simulink model "systema2011a"  (Simulink 7.7)
settings: Solver=ode4  StartTime=0.0  StopTime=20  FixedStep=0.01  RelTol=1e-3
libraries: simulink x11
CloseFcn:
  | rtwprivate ssgencode ModelCloseRequest systema
settings Model: Creator=ece  LastModifiedBy=lenovo
settings DataIOCC: LimitDataPoints=off  SignalLoggingSaveFormat=Dataset  SignalLoggingName=sigsOut
settings OptimizationCC: OptimizeBlockIOStorage=off  BufferReuse=off  ExpressionFolding=off  LocalBlockOutputs=off  InitFltsAndDblsToZero=on
settings DebuggingCC: SaveWithParameterizedLinksMsg=none  SignalResolutionControl=TryResolveAllWithWarning  SolverPrmCheckMsg=none  MultiTaskDSMMsg=warning  MultiTaskCondExecSysMsg=none  FcnCallInpInsideContextMsg=Enable All
settings HardwareCC: TargetUnknown=on
settings CodeAppCC: CustomSymbolStrType=$N$R$M_T
settings GRTTargetCC: TargetFcnLib=ansi_tfl_tmw.mat  TargetFunctionLibrary=C89/C90 (ANSI)  ModelReferenceCompliant=off  MatFileLogging=off

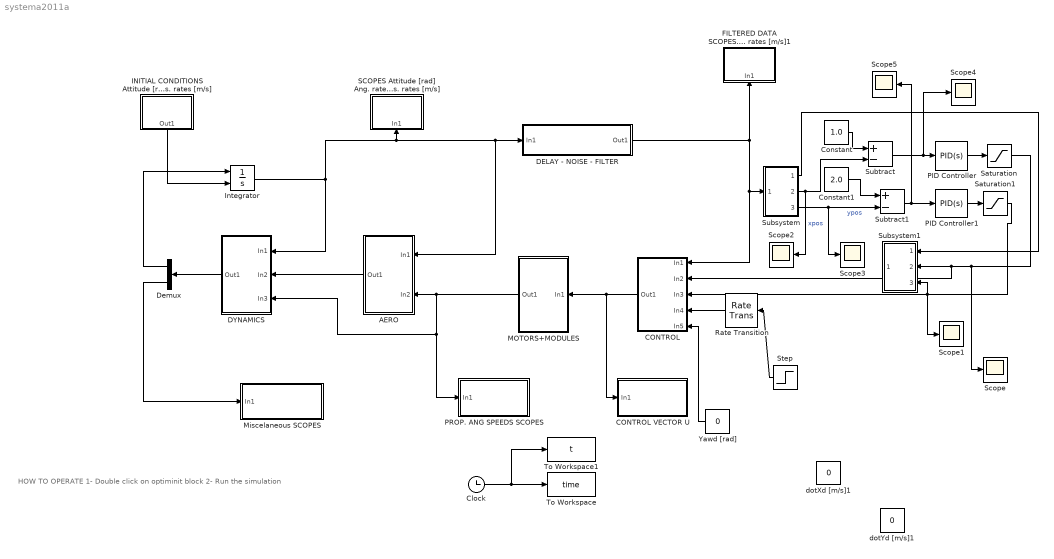
== system systema2011a ==
  note: HOW TO OPERATE
      | 1- Double click on optiminit block
      | 2- Run the simulation
  AERO : Subsystem
  CONTROL : Subsystem
  CONTROL VECTOR U : Subsystem
  Clock : Clock
  Constant : Constant  Value=1.0
  Constant1 : Constant  Value=2.0
  DELAY - NOISE - FILTER : Subsystem
  DYNAMICS : Subsystem
  Demux : Demux  Outputs=2
  FILTERED DATA SCOPES Attitude [rad] Ang. rates [rad/sec] position [m] Pos. rates [m/s]1 : Subsystem
  "INITIAL CONDITIONS Attitude [rad] Ang. rates [rad/sec] position [m] Pos. rates [m/s] " : Subsystem
  Integrator : Integrator  InitialConditionSource=external
  MOTORS+MODULES : Subsystem
  Miscelaneous SCOPES : Subsystem
  PID Controller : simulink/Continuous/PID Controller  Controller=PID  TimeDomain=Continuous-time  SampleTime=-1  IntegratorMethod=Forward Euler  FilterMethod=Forward Euler  Form=Parallel  UseFilter=on  ControllerParametersSource=internal  P=0.8  I=0.2  D=0  N=100  InitialConditionSource=internal  InitialConditionForIntegrator=0  InitialConditionForFilter=0  ExternalReset=none  LimitOutput=off  UpperSaturationLimit=inf  LowerSaturationLimit=-inf  LinearizeAsGain=off  AntiWindupMode=none  Kb=1  TrackingMode=off  Kt=1  PParamMin=[]  PParamMax=[]  IParamMin=[]  IParamMax=[]  DParamMin=[]  DParamMax=[]  NParamMin=[]  NParamMax=[]  KbParamMin=[]  KbParamMax=[]  KtParamMin=[]  KtParamMax=[]  POutMin=[]  POutMax=[]  IOutMin=[]  IOutMax=[]  DOutMin=[]  DOutMax=[]  NOutMin=[]  NOutMax=[]  KbOutMin=[]  KbOutMax=[]  KtOutMin=[]  KtOutMax=[]  IntegratorOutMin=[]  IntegratorOutMax=[]  FilterOutMin=[]  FilterOutMax=[]  SumOutMin=[]  SumOutMax=[]  SumI1OutMin=[]  SumI1OutMax=[]  SumI2OutMin=[]  SumI2OutMax=[]  SumI3OutMin=[]  SumI3OutMax=[]  SumDOutMin=[]  SumDOutMax=[]  SaturationOutMin=[]  SaturationOutMax=[]  IntegratorContinuousStateAttributes=''  IntegratorStateMustResolveToSignalObject=off  IntegratorRTWStateStorageClass=Auto  FilterContinuousStateAttributes=''  FilterStateMustResolveToSignalObject=off  FilterRTWStateStorageClass=Auto  DifferentiatorICPrevScaledInput=0  DifferentiatorOutMin=[]  DifferentiatorOutMax=[]
  PID Controller1 : simulink/Continuous/PID Controller  Controller=PID  TimeDomain=Continuous-time  SampleTime=-1  IntegratorMethod=Forward Euler  FilterMethod=Forward Euler  Form=Parallel  UseFilter=on  ControllerParametersSource=internal  P=1  I=0.2  D=0  N=100  InitialConditionSource=internal  InitialConditionForIntegrator=0  InitialConditionForFilter=0  ExternalReset=none  LimitOutput=off  UpperSaturationLimit=inf  LowerSaturationLimit=-inf  LinearizeAsGain=off  AntiWindupMode=none  Kb=1  TrackingMode=off  Kt=1  PParamMin=[]  PParamMax=[]  IParamMin=[]  IParamMax=[]  DParamMin=[]  DParamMax=[]  NParamMin=[]  NParamMax=[]  KbParamMin=[]  KbParamMax=[]  KtParamMin=[]  KtParamMax=[]  POutMin=[]  POutMax=[]  IOutMin=[]  IOutMax=[]  DOutMin=[]  DOutMax=[]  NOutMin=[]  NOutMax=[]  KbOutMin=[]  KbOutMax=[]  KtOutMin=[]  KtOutMax=[]  IntegratorOutMin=[]  IntegratorOutMax=[]  FilterOutMin=[]  FilterOutMax=[]  SumOutMin=[]  SumOutMax=[]  SumI1OutMin=[]  SumI1OutMax=[]  SumI2OutMin=[]  SumI2OutMax=[]  SumI3OutMin=[]  SumI3OutMax=[]  SumDOutMin=[]  SumDOutMax=[]  SaturationOutMin=[]  SaturationOutMax=[]  IntegratorContinuousStateAttributes=''  IntegratorStateMustResolveToSignalObject=off  IntegratorRTWStateStorageClass=Auto  FilterContinuousStateAttributes=''  FilterStateMustResolveToSignalObject=off  FilterRTWStateStorageClass=Auto  DifferentiatorICPrevScaledInput=0  DifferentiatorOutMin=[]  DifferentiatorOutMax=[]
  PROP. ANG SPEEDS SCOPES : Subsystem
  Rate Transition : RateTransition
  SCOPES Attitude [rad] Ang. rates [rad/sec] position [m] Pos. rates [m/s] : Subsystem
  Saturation : Saturate  UpperLimit=20  LowerLimit=-20
  Saturation1 : Saturate  UpperLimit=20  LowerLimit=-20
  Scope{,1..5} (6 alike) : Scope
      Scope settings: TimeRange=auto  LimitDataPoints=on  MaxDataPoints=5000  SaveToWorkspace=off  SaveName=ScopeData13  YMin=-50  YMax=400  SampleTime=-1
      Scope1 settings: TimeRange=auto  LimitDataPoints=on  MaxDataPoints=5000  SaveToWorkspace=off  SaveName=ScopeData19  YMin=75  YMax=400  SampleTime=-1
      Scope2 settings: TimeRange=auto  LimitDataPoints=on  MaxDataPoints=5000  SaveToWorkspace=off  SaveName=ScopeData28  YMin=-0.16677  YMax=1.5009  SampleTime=-1
      Scope3 settings: TimeRange=auto  LimitDataPoints=on  MaxDataPoints=5000  SaveToWorkspace=off  SaveName=ScopeData29  YMin=-1.59858  YMax=3.92406  SampleTime=-1
      Scope4 settings: TimeRange=auto  LimitDataPoints=on  MaxDataPoints=5000  SaveToWorkspace=off  SaveName=ScopeData30  YMin=75  YMax=400  SampleTime=-1
      Scope5 settings: TimeRange=auto  LimitDataPoints=on  MaxDataPoints=5000  SaveToWorkspace=off  SaveName=ScopeData31  YMin=75  YMax=400  SampleTime=-1
  Step : Step  Time=10  Before=3  After=3.5  SampleTime=0
  Subsystem : Subsystem
  Subsystem1 : Subsystem
  Subtract : Sum  Inputs=+-
  Subtract1 : Sum  Inputs=+-
  To Workspace : ToWorkspace  VariableName=time  SampleTime=-1
  To Workspace1 : ToWorkspace  VariableName=t  SampleTime=-1
  Yawd [rad] : Constant  Value=0
  dotXd [m/s]1 : Constant  Value=0
  dotYd [m/s]1 : Constant  Value=0
  wires:
  Integrator/1 -> SCOPES Attitude [rad] Ang. rates [rad/sec] position [m] Pos. rates [m/s]/1(In1), DELAY - NOISE - FILTER/1(In1), AERO/1(In1), DYNAMICS/1(In1)
  "INITIAL CONDITIONS Attitude [rad] Ang. rates [rad/sec] position [m] Pos. rates [m/s] "/1(Out1) -> Integrator/2
  Clock/1 -> To Workspace/1, To Workspace1/1
  DYNAMICS/1(Out1) -> Demux/1
  Demux/1 -> Integrator/1
  Demux/2 -> Miscelaneous SCOPES/1(In1)
  CONTROL/1(Out1) -> MOTORS+MODULES/1(In1), CONTROL VECTOR U/1(In1)
  Yawd [rad]/1 -> CONTROL/5(In5)
  MOTORS+MODULES/1(Out1) -> AERO/2(In2), DYNAMICS/3(In3), PROP. ANG SPEEDS SCOPES/1(In1)
  AERO/1(Out1) -> DYNAMICS/2(In2)
  DELAY - NOISE - FILTER/1(Out1) -> FILTERED DATA SCOPES Attitude [rad] Ang. rates [rad/sec] position [m] Pos. rates [m/s]1/1(In1), CONTROL/1(In1), Subsystem/1(In1)
  Subtract/1 -> PID Controller/1, Scope4/1
  Subtract1/1 -> PID Controller1/1, Scope5/1
  Subsystem/2(Out3) -> Subtract/2, Scope2/1  "xpos"
  Subsystem/3(Out4) -> Subtract1/2, Scope3/1  "ypos"
  Constant/1 -> Subtract/1
  Constant1/1 -> Subtract1/1
  Subsystem/1(Out2) -> Subsystem1/1(In1)
  PID Controller1/1 -> Saturation1/1
  PID Controller/1 -> Saturation/1
  Saturation/1 -> Scope/1, Subsystem1/2(In2), CONTROL/2(In2)
  Saturation1/1 -> CONTROL/3(In3), Subsystem1/3(In3), Scope1/1
  Rate Transition/1 -> CONTROL/4(In4)
  Step/1 -> Rate Transition/1

== system systema2011a/AERO ==
  In1 : Inport
  In2 : Inport  Port=2
  AERO Attitude [rad] : MATLABFcn  MATLABFcn=aero  OutputDimensions=24
  Mux1 : Mux  Inputs=2
  Out1 : Outport
  wires:
  In1/1 -> Mux1/1
  In2/1 -> Mux1/2
  Mux1/1 -> AERO Attitude [rad]/1
  AERO Attitude [rad]/1 -> Out1/1

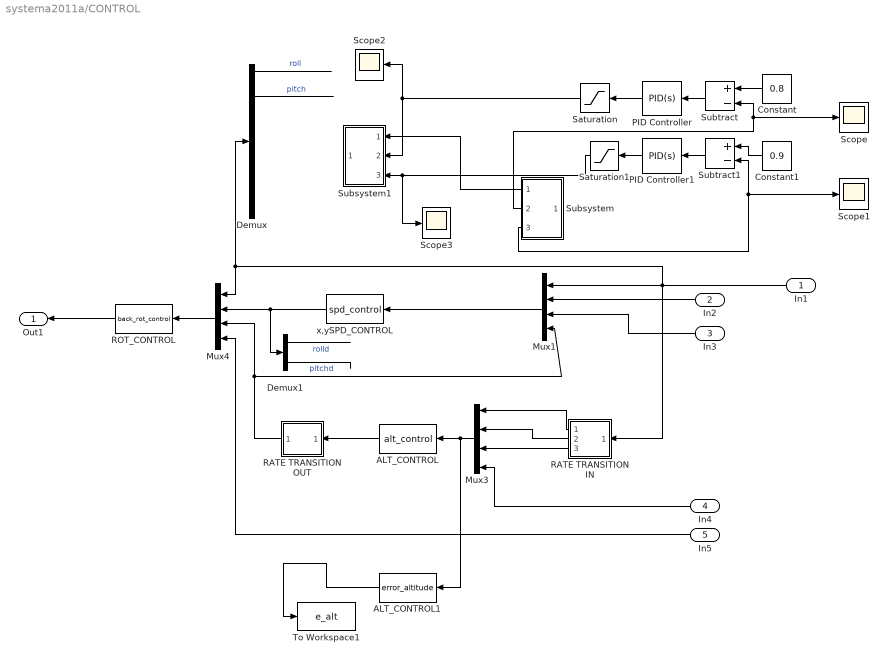
== system systema2011a/CONTROL ==
  In1 : Inport
  In2 : Inport  Port=2
  In3 : Inport  Port=3
  In4 : Inport  Port=4
  In5 : Inport  Port=5
  ALT_CONTROL : MATLABFcn  MATLABFcn=alt_control  OutputDimensions=1  SampleTime=0.05
  ALT_CONTROL1 : MATLABFcn  MATLABFcn=error_altitude  OutputDimensions=1  SampleTime=0.05
  Constant : Constant  Value=0.8
  Constant1 : Constant  Value=0.9
  Demux : Demux  Outputs=12
  Demux1 : Demux  Outputs=2
  Mux1 : Mux
  Mux3 : Mux
  Mux4 : Mux
  PID Controller : simulink/Continuous/PID Controller  Controller=PID  TimeDomain=Continuous-time  SampleTime=-1  IntegratorMethod=Forward Euler  FilterMethod=Forward Euler  Form=Parallel  UseFilter=on  ControllerParametersSource=internal  P=10  I=0.01  D=2  N=100  InitialConditionSource=internal  InitialConditionForIntegrator=0  InitialConditionForFilter=0  ExternalReset=none  LimitOutput=off  UpperSaturationLimit=inf  LowerSaturationLimit=-inf  LinearizeAsGain=off  AntiWindupMode=none  Kb=1  TrackingMode=off  Kt=1  PParamMin=[]  PParamMax=[]  IParamMin=[]  IParamMax=[]  DParamMin=[]  DParamMax=[]  NParamMin=[]  NParamMax=[]  KbParamMin=[]  KbParamMax=[]  KtParamMin=[]  KtParamMax=[]  POutMin=[]  POutMax=[]  IOutMin=[]  IOutMax=[]  DOutMin=[]  DOutMax=[]  NOutMin=[]  NOutMax=[]  KbOutMin=[]  KbOutMax=[]  KtOutMin=[]  KtOutMax=[]  IntegratorOutMin=[]  IntegratorOutMax=[]  FilterOutMin=[]  FilterOutMax=[]  SumOutMin=[]  SumOutMax=[]  SumI1OutMin=[]  SumI1OutMax=[]  SumI2OutMin=[]  SumI2OutMax=[]  SumI3OutMin=[]  SumI3OutMax=[]  SumDOutMin=[]  SumDOutMax=[]  SaturationOutMin=[]  SaturationOutMax=[]  IntegratorContinuousStateAttributes=''  IntegratorStateMustResolveToSignalObject=off  IntegratorRTWStateStorageClass=Auto  FilterContinuousStateAttributes=''  FilterStateMustResolveToSignalObject=off  FilterRTWStateStorageClass=Auto  DifferentiatorICPrevScaledInput=0  DifferentiatorOutMin=[]  DifferentiatorOutMax=[]
  PID Controller1 : simulink/Continuous/PID Controller  Controller=PID  TimeDomain=Continuous-time  SampleTime=-1  IntegratorMethod=Forward Euler  FilterMethod=Forward Euler  Form=Parallel  UseFilter=on  ControllerParametersSource=internal  P=10  I=0.01  D=3  N=100  InitialConditionSource=internal  InitialConditionForIntegrator=0  InitialConditionForFilter=0  ExternalReset=none  LimitOutput=off  UpperSaturationLimit=inf  LowerSaturationLimit=-inf  LinearizeAsGain=off  AntiWindupMode=none  Kb=1  TrackingMode=off  Kt=1  PParamMin=[]  PParamMax=[]  IParamMin=[]  IParamMax=[]  DParamMin=[]  DParamMax=[]  NParamMin=[]  NParamMax=[]  KbParamMin=[]  KbParamMax=[]  KtParamMin=[]  KtParamMax=[]  POutMin=[]  POutMax=[]  IOutMin=[]  IOutMax=[]  DOutMin=[]  DOutMax=[]  NOutMin=[]  NOutMax=[]  KbOutMin=[]  KbOutMax=[]  KtOutMin=[]  KtOutMax=[]  IntegratorOutMin=[]  IntegratorOutMax=[]  FilterOutMin=[]  FilterOutMax=[]  SumOutMin=[]  SumOutMax=[]  SumI1OutMin=[]  SumI1OutMax=[]  SumI2OutMin=[]  SumI2OutMax=[]  SumI3OutMin=[]  SumI3OutMax=[]  SumDOutMin=[]  SumDOutMax=[]  SaturationOutMin=[]  SaturationOutMax=[]  IntegratorContinuousStateAttributes=''  IntegratorStateMustResolveToSignalObject=off  IntegratorRTWStateStorageClass=Auto  FilterContinuousStateAttributes=''  FilterStateMustResolveToSignalObject=off  FilterRTWStateStorageClass=Auto  DifferentiatorICPrevScaledInput=0  DifferentiatorOutMin=[]  DifferentiatorOutMax=[]
  RATE TRANSITION IN : Subsystem
  RATE TRANSITION OUT : Subsystem
  ROT_CONTROL : MATLABFcn  MATLABFcn=back_rot_control  OutputDimensions=6
  Saturation : Saturate  UpperLimit=20  LowerLimit=-20
  Saturation1 : Saturate  UpperLimit=20  LowerLimit=-20
  Scope{,1..3} (4 alike) : Scope
      Scope settings: TimeRange=auto  LimitDataPoints=on  MaxDataPoints=5000  SaveToWorkspace=off  SaveName=ScopeData20  YMin=-0.5  YMax=2  SampleTime=-1
      Scope1 settings: TimeRange=auto  LimitDataPoints=on  MaxDataPoints=5000  SaveToWorkspace=off  SaveName=ScopeData21  YMin=-50  YMax=400  SampleTime=-1
      Scope2 settings: TimeRange=auto  LimitDataPoints=on  MaxDataPoints=5000  SaveToWorkspace=off  SaveName=ScopeData22  YMin=-50  YMax=400  SampleTime=-1
      Scope3 settings: TimeRange=auto  LimitDataPoints=on  MaxDataPoints=5000  SaveToWorkspace=off  SaveName=ScopeData23  YMin=-50  YMax=400  SampleTime=-1
  Subsystem : Subsystem
  Subsystem1 : Subsystem
  Subtract : Sum  Inputs=+-
  Subtract1 : Sum  Inputs=+-
  To Workspace1 : ToWorkspace  VariableName=e_alt  SampleTime=-1
  x,ySPD_CONTROL : MATLABFcn  MATLABFcn=spd_control  OutputDimensions=2
  Out1 : Outport
  wires:
  Mux1/1 -> x,ySPD_CONTROL/1
  ROT_CONTROL/1 -> Out1/1
  In1/1 -> Mux1/1, RATE TRANSITION IN/1(In1), Demux/1, Mux4/1
  In2/1 -> Mux1/2
  x,ySPD_CONTROL/1 -> Demux1/1, Mux4/2
  Mux4/1 -> ROT_CONTROL/1
  ALT_CONTROL/1 -> RATE TRANSITION OUT/1(In1)
  In5/1 -> Mux4/4
  RATE TRANSITION OUT/1(Out1) -> Mux4/3, Mux1/4
  Mux3/1 -> ALT_CONTROL/1, ALT_CONTROL1/1
  RATE TRANSITION IN/1(Out1) -> Mux3/1
  RATE TRANSITION IN/2(Out2) -> Mux3/2
  RATE TRANSITION IN/3(Out3) -> Mux3/3
  In4/1 -> Mux3/4
  In3/1 -> Mux1/3
  ALT_CONTROL1/1 -> To Workspace1/1
  Subtract/1 -> PID Controller/1
  Subtract1/1 -> PID Controller1/1
  Constant/1 -> Subtract/1
  Constant1/1 -> Subtract1/1
  PID Controller1/1 -> Saturation1/1
  PID Controller/1 -> Saturation/1
  Subsystem/1(Out2) -> Subsystem1/1(In1)
  Subsystem/2(Out3) -> Subtract/2, Scope/1
  Subsystem/3(Out4) -> Subtract1/2, Scope1/1
  Saturation/1 -> Subsystem1/2(In2), Scope2/1
  Saturation1/1 -> Subsystem1/3(In3), Scope3/1
  Demux/1 -> ?  "roll"
  Demux/3 -> ?  "pitch"
  Demux1/1 -> ?  "rolld"
  Demux1/2 -> ?  "pitchd"

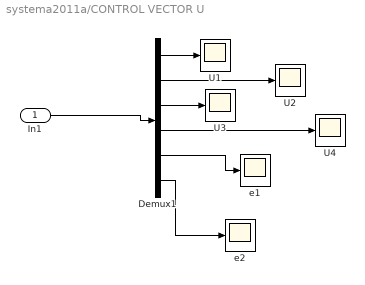
== system systema2011a/CONTROL VECTOR U ==
  In1 : Inport
  Demux1 : Demux  Outputs=6
  U{1..4} (4 alike) : Scope
      U1 settings: TimeRange=3.5  MaxDataPoints=5000  SaveToWorkspace=off  SaveName=ScopeData7  YMin=144.101  YMax=144.104  SampleTime=-1
      U2 settings: TimeRange=auto  MaxDataPoints=5000  SaveToWorkspace=off  SaveName=ScopeData8  YMin=-0.6  YMax=0.4  SampleTime=-1
      U3 settings: TimeRange=auto  MaxDataPoints=5000  SaveToWorkspace=off  SaveName=ScopeData9  YMin=-0.65  YMax=0.35  SampleTime=-1
      U4 settings: TimeRange=auto  MaxDataPoints=5000  SaveToWorkspace=off  SaveName=ScopeData14  YMin=0  YMax=150  SampleTime=-1
  e1 : Scope
      settings: TimeRange=auto  MaxDataPoints=5000  SaveToWorkspace=off  SaveName=ScopeData11  YMin=0  YMax=150  SampleTime=-1
  e2 : Scope
      settings: TimeRange=auto  MaxDataPoints=5000  SaveToWorkspace=off  SaveName=ScopeData12  YMin=0  YMax=150  SampleTime=-1
  wires:
  In1/1 -> Demux1/1
  Demux1/4 -> U4/1
  Demux1/3 -> U3/1
  Demux1/2 -> U2/1
  Demux1/1 -> U1/1
  Demux1/5 -> e1/1
  Demux1/6 -> e2/1

== system systema2011a/DELAY - NOISE - FILTER ==
  In1 : Inport
  DELAYS : Subsystem
  LP FILTER : MATLABFcn  MATLABFcn=sam5_filter  OutputDimensions=12  OutputSignalType=real
  NOISY DATA SCOPES Attitude [rad] Ang. rates [rad/sec] position [m] Pos. rates [m/s]1 : Subsystem
  W. NORMAL NOISE1 : Subsystem
  Out1 : Outport
  wires:
  In1/1 -> DELAYS/1(In1)
  DELAYS/1(Out1) -> NOISY DATA SCOPES Attitude [rad] Ang. rates [rad/sec] position [m] Pos. rates [m/s]1/1(In1), LP FILTER/1
  LP FILTER/1 -> Out1/1

== system systema2011a/DYNAMICS ==
  In1 : Inport
  In2 : Inport  Port=2
  In3 : Inport  Port=3
  DYNAMICS : MATLABFcn  MATLABFcn=dinamica  OutputDimensions=18
  Mux1 : Mux  Inputs=3
  Out1 : Outport
  wires:
  DYNAMICS/1 -> Out1/1
  Mux1/1 -> DYNAMICS/1
  In2/1 -> Mux1/2
  In1/1 -> Mux1/1
  In3/1 -> Mux1/3

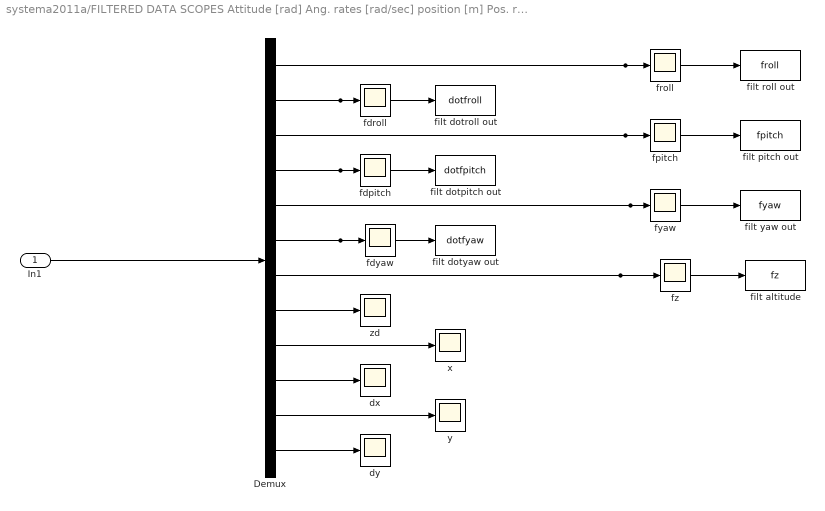
== system systema2011a/FILTERED DATA SCOPES Attitude [rad] Ang. rates [rad/sec] position [m] Pos. rates [m/s]1 ==
  In1 : Inport
  Demux : Demux  Outputs=12
  dx : Scope
      settings: TimeRange=5  MaxDataPoints=5000  SaveToWorkspace=off  SaveName=ScopeData5  YMin=0  YMax=0.009  SampleTime=-1
  dy : Scope
      settings: TimeRange=5  MaxDataPoints=5000  SaveToWorkspace=off  SaveName=ScopeData10  YMin=0  YMax=0.009  SampleTime=-1
  fdpitch : Scope
      settings: TimeRange=auto  MaxDataPoints=5000  SaveToWorkspace=off  SaveName=ScopeData15  YMin=-2250  YMax=2250  SampleTime=-1
  fdroll : Scope
      settings: TimeRange=auto  MaxDataPoints=5000  SaveToWorkspace=off  SaveName=ScopeData14  YMin=-0.25  YMax=-0.05  SampleTime=-1
  fdyaw : Scope
      settings: TimeRange=18  MaxDataPoints=5000  SaveToWorkspace=off  SaveName=ScopeData16  YMin=-200  YMax=200  SampleTime=-1
  filt altitude : ToWorkspace  VariableName=fz  SampleTime=-1
  filt dotpitch out : ToWorkspace  VariableName=dotfpitch  SampleTime=-1
  filt dotroll out : ToWorkspace  VariableName=dotfroll  SampleTime=-1
  filt dotyaw out : ToWorkspace  VariableName=dotfyaw  SampleTime=-1
  filt pitch out : ToWorkspace  VariableName=fpitch  SampleTime=-1
  filt roll out : ToWorkspace  VariableName=froll  SampleTime=-1
  filt yaw out : ToWorkspace  VariableName=fyaw  SampleTime=-1
  fpitch : Scope
      settings: TimeRange=4  MaxDataPoints=5000  SaveToWorkspace=off  YMin=-1  YMax=1  SampleTime=-1
  froll : Scope
      settings: TimeRange=0.25  MaxDataPoints=5000  SaveToWorkspace=off  SaveName=ScopeData  YMin=-1  YMax=1  SampleTime=-1
  fyaw : Scope
      settings: TimeRange=5  MaxDataPoints=5000  SaveToWorkspace=off  SaveName=ScopeData2  YMin=0  YMax=0.22  SampleTime=-1
  fz : Scope
      settings: TimeRange=5  MaxDataPoints=5000  SaveToWorkspace=off  SaveName=ScopeData17  YMin=-0.45  YMax=0.5  SampleTime=-1
  x : Scope
      settings: TimeRange=5  MaxDataPoints=5000  SaveToWorkspace=off  SaveName=ScopeData4  YMin=0  YMax=0.009  SampleTime=-1
  y : Scope
      settings: TimeRange=5  MaxDataPoints=5000  SaveToWorkspace=off  SaveName=ScopeData6  YMin=0  YMax=0.009  SampleTime=-1
  zd : Scope
      settings: TimeRange=10  MaxDataPoints=5000  SaveToWorkspace=off  SaveName=ScopeData18  YMin=-110.5  YMax=-107.25  SampleTime=-1
  wires:
  Demux/1 -> filt roll out/1, froll/1
  Demux/4 -> fdpitch/1, filt dotpitch out/1
  Demux/8 -> zd/1
  Demux/7 -> filt altitude/1, fz/1
  Demux/6 -> fdyaw/1, filt dotyaw out/1
  Demux/2 -> fdroll/1, filt dotroll out/1
  Demux/5 -> filt yaw out/1, fyaw/1
  Demux/3 -> filt pitch out/1, fpitch/1
  In1/1 -> Demux/1
  Demux/9 -> x/1
  Demux/10 -> dx/1
  Demux/11 -> y/1
  Demux/12 -> dy/1

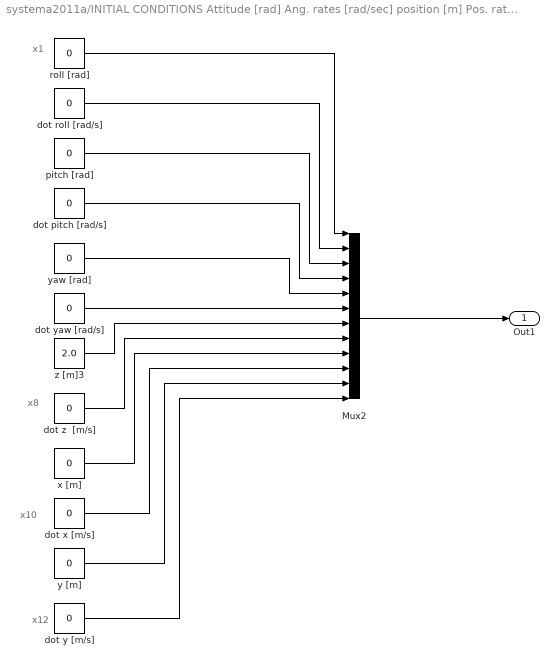
== system systema2011a/INITIAL CONDITIONS Attitude [rad] Ang. rates [rad/sec] position [m] Pos. rates [m/s]  ==
  note: x1
  note: x12
  note: x10
  note: x8
  Mux2 : Mux  Inputs=12
  dot pitch [rad/s] : Constant  Value=0
  dot roll [rad/s] : Constant  Value=0
  dot x [m/s] : Constant  Value=0
  dot y [m/s] : Constant  Value=0
  dot yaw [rad/s] : Constant  Value=0
  dot z  [m/s] : Constant  Value=0
  pitch [rad] : Constant  Value=0
  roll [rad] : Constant  Value=0
  x [m] : Constant  Value=0
  y [m] : Constant  Value=0
  yaw [rad] : Constant  Value=0
  z [m]3 : Constant  Value=2.0
  Out1 : Outport
  wires:
  roll [rad]/1 -> Mux2/1
  dot roll [rad/s]/1 -> Mux2/2
  pitch [rad]/1 -> Mux2/3
  dot pitch [rad/s]/1 -> Mux2/4
  dot yaw [rad/s]/1 -> Mux2/6
  z [m]3/1 -> Mux2/7
  dot z  [m/s]/1 -> Mux2/8
  yaw [rad]/1 -> Mux2/5
  Mux2/1 -> Out1/1
  x [m]/1 -> Mux2/9
  dot x [m/s]/1 -> Mux2/10
  y [m]/1 -> Mux2/11
  dot y [m/s]/1 -> Mux2/12

== system systema2011a/MOTORS+MODULES ==
  In1 : Inport
  Bin2Om : MATLABFcn  MATLABFcn=bin2Om  OutputDimensions=4  OutputSignalType=real
  MOTOR DYNAMICS : Subsystem
  Saturation : Saturate  UpperLimit=125  LowerLimit=10
  U2bin : MATLABFcn  MATLABFcn=U2bin  OutputDimensions=4  OutputSignalType=real
  Out1 : Outport
  wires:
  Bin2Om/1 -> Out1/1
  MOTOR DYNAMICS/1(Out1) -> Bin2Om/1
  U2bin/1 -> Saturation/1
  In1/1 -> U2bin/1
  Saturation/1 -> MOTOR DYNAMICS/1(In1)

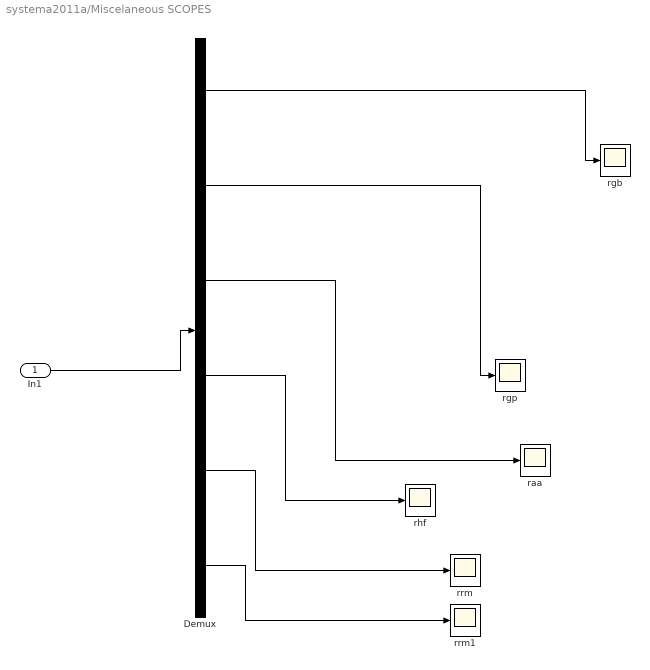
== system systema2011a/Miscelaneous SCOPES ==
  In1 : Inport  PortDimensions=6
  Demux : Demux  Outputs=6
  raa : Scope
      settings: TimeRange=18  MaxDataPoints=5000  SaveToWorkspace=off  SaveName=ScopeData16  YMin=-200  YMax=200  SampleTime=-1
  rgb : Scope
      settings: TimeRange=auto  MaxDataPoints=5000  SaveToWorkspace=off  SaveName=ScopeData14  YMin=-0.25  YMax=-0.05  SampleTime=-1
  rgp : Scope
      settings: TimeRange=auto  MaxDataPoints=5000  SaveToWorkspace=off  SaveName=ScopeData15  YMin=-2250  YMax=2250  SampleTime=-1
  rhf : Scope
      settings: TimeRange=10  MaxDataPoints=5000  SaveToWorkspace=off  SaveName=ScopeData18  YMin=-110.5  YMax=-107.25  SampleTime=-1
  rrm : Scope
      settings: TimeRange=5  MaxDataPoints=5000  SaveToWorkspace=off  SaveName=ScopeData25  YMin=-4.75e-015  YMax=0  SampleTime=-1
  rrm1 : Scope
      settings: TimeRange=5  MaxDataPoints=5000  SaveToWorkspace=off  SaveName=ScopeData3  YMin=-4.75e-015  YMax=0  SampleTime=-1
  wires:
  In1/1 -> Demux/1
  Demux/5 -> rrm/1
  Demux/4 -> rhf/1
  Demux/3 -> raa/1
  Demux/2 -> rgp/1
  Demux/1 -> rgb/1
  Demux/6 -> rrm1/1

== system systema2011a/PROP. ANG SPEEDS SCOPES ==
  In1 : Inport
  Demux1 : Demux
  omega{1..4} (4 alike) : Scope
      omega1 settings: TimeRange=3.5  MaxDataPoints=5000  SaveToWorkspace=off  SaveName=ScopeData7  YMin=144.101  YMax=144.104  SampleTime=-1
      omega2 settings: TimeRange=auto  MaxDataPoints=5000  SaveToWorkspace=off  SaveName=ScopeData8  YMin=142.5  YMax=147.5  SampleTime=-1
      omega3 settings: TimeRange=auto  MaxDataPoints=5000  SaveToWorkspace=off  SaveName=ScopeData9  YMin=0  YMax=150  SampleTime=-1
      omega4 settings: TimeRange=auto  MaxDataPoints=5000  SaveToWorkspace=off  SaveName=ScopeData14  YMin=0  YMax=150  SampleTime=-1
  wires:
  Demux1/1 -> omega1/1
  Demux1/2 -> omega2/1
  Demux1/3 -> omega3/1
  Demux1/4 -> omega4/1
  In1/1 -> Demux1/1

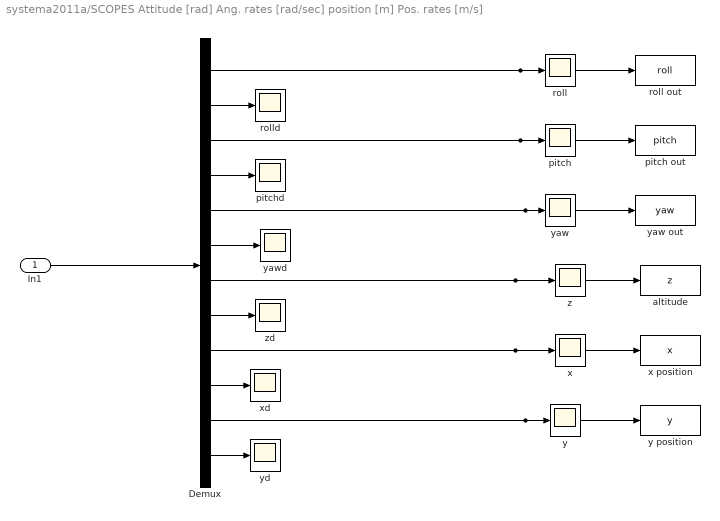
== system systema2011a/SCOPES Attitude [rad] Ang. rates [rad/sec] position [m] Pos. rates [m/s] ==
  In1 : Inport
  Demux : Demux  Outputs=12
  altitude : ToWorkspace  VariableName=z  SampleTime=-1
  pitch : Scope
      settings: TimeRange=4  MaxDataPoints=5000  SaveToWorkspace=off  YMin=-0.08  YMax=0.16  SampleTime=-1
  pitch out : ToWorkspace  VariableName=pitch  SampleTime=-1
  pitchd : Scope
      settings: TimeRange=auto  MaxDataPoints=5000  SaveToWorkspace=off  SaveName=ScopeData15  YMin=-1.75  YMax=1.75  SampleTime=-1
  roll : Scope
      settings: TimeRange=0.25  MaxDataPoints=5000  SaveToWorkspace=off  SaveName=ScopeData  YMin=-0.008  YMax=0.005  SampleTime=-1
  roll out : ToWorkspace  VariableName=roll  SampleTime=-1
  rolld : Scope
      settings: TimeRange=7  MaxDataPoints=5000  SaveToWorkspace=off  SaveName=ScopeData14  YMin=-0.15  YMax=0.125  SampleTime=-1
  x : Scope
      settings: TimeRange=5  MaxDataPoints=5000  SaveToWorkspace=off  SaveName=ScopeData24  YMin=-1  YMax=1  SampleTime=-1
  x position : ToWorkspace  VariableName=x  SampleTime=-1
  xd : Scope
      settings: TimeRange=5  MaxDataPoints=5000  SaveToWorkspace=off  SaveName=ScopeData25  YMin=-4.75e-015  YMax=0  SampleTime=-1
  y : Scope
      settings: TimeRange=5  MaxDataPoints=5000  SaveToWorkspace=off  SaveName=ScopeData26  YMin=-1  YMax=1  SampleTime=-1
  y position : ToWorkspace  VariableName=y  SampleTime=-1
  yaw : Scope
      settings: TimeRange=5  MaxDataPoints=5000  SaveToWorkspace=off  SaveName=ScopeData2  YMin=-175  YMax=0  SampleTime=-1
  yaw out : ToWorkspace  VariableName=yaw  SampleTime=-1
  yawd : Scope
      settings: TimeRange=18  MaxDataPoints=5000  SaveToWorkspace=off  SaveName=ScopeData16  YMin=-0.275  YMax=0.15  SampleTime=-1
  yd : Scope
      settings: TimeRange=5  MaxDataPoints=5000  SaveToWorkspace=off  SaveName=ScopeData27  YMin=-143.75  YMax=-141.75  SampleTime=-1
  z : Scope
      settings: TimeRange=5  MaxDataPoints=5000  SaveToWorkspace=off  SaveName=ScopeData17  YMin=0  YMax=0.009  SampleTime=-1
  zd : Scope
      settings: TimeRange=10  MaxDataPoints=5000  SaveToWorkspace=off  SaveName=ScopeData18  YMin=-110.5  YMax=-107.25  SampleTime=-1
  wires:
  In1/1 -> Demux/1
  Demux/3 -> pitch/1, pitch out/1
  Demux/5 -> yaw/1, yaw out/1
  Demux/2 -> rolld/1
  Demux/6 -> yawd/1
  Demux/7 -> z/1, altitude/1
  Demux/8 -> zd/1
  Demux/9 -> x/1, x position/1
  Demux/11 -> y/1, y position/1
  Demux/12 -> yd/1
  Demux/10 -> xd/1
  Demux/4 -> pitchd/1
  Demux/1 -> roll/1, roll out/1

== system systema2011a/Subsystem ==
  In1 : Inport
  Demux1 : Demux  Outputs=12
  Double click on this for demo.5 : Subsystem
      settings: OpenFcn=optsiminit
      mask Display: disp('optsiminit')
  Mux1 : Mux  Inputs=10
  Out2 : Outport
  Out3 : Outport  Port=2
  Out4 : Outport  Port=3
  wires:
  Demux1/1 -> Mux1/1
  Demux1/2 -> Mux1/2
  Demux1/3 -> Mux1/3
  Demux1/4 -> Mux1/4
  Demux1/5 -> Mux1/5
  Demux1/6 -> Mux1/6
  Demux1/7 -> Mux1/7
  Demux1/8 -> Mux1/8
  Demux1/10 -> Mux1/9
  Demux1/12 -> Mux1/10
  Mux1/1 -> Out2/1
  Demux1/9 -> Out3/1
  Demux1/11 -> Out4/1
  In1/1 -> Demux1/1

== system systema2011a/Subsystem1 ==
  In1 : Inport
  In2 : Inport  Port=2
  In3 : Inport  Port=3
  Demux1 : Demux  Outputs=10
  Mux1 : Mux  Inputs=12
  Out5 : Outport
  wires:
  In1/1 -> Demux1/1
  Demux1/1 -> Mux1/1
  Demux1/2 -> Mux1/2
  Demux1/3 -> Mux1/3
  Demux1/4 -> Mux1/4
  Demux1/5 -> Mux1/5
  Demux1/6 -> Mux1/6
  Demux1/7 -> Mux1/7
  Demux1/8 -> Mux1/8
  Demux1/10 -> Mux1/12
  Demux1/9 -> Mux1/10
  In2/1 -> Mux1/9
  In3/1 -> Mux1/11
  Mux1/1 -> Out5/1

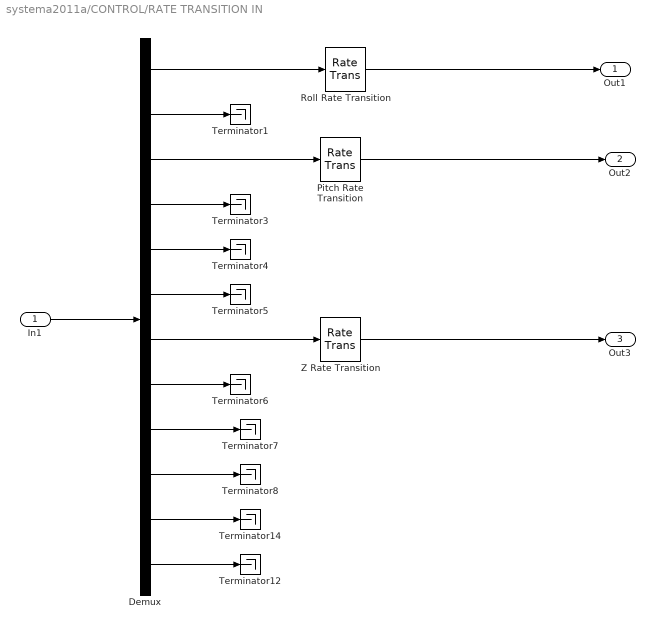
== system systema2011a/CONTROL/RATE TRANSITION IN ==
  In1 : Inport
  Demux : Demux  Outputs=12
  Pitch Rate Transition : RateTransition  Deterministic=off  OutPortSampleTime=50E-3
  Roll Rate Transition : RateTransition  Deterministic=off  OutPortSampleTime=50E-3
  Terminator{1,3..8,12,14} (9 alike) : Terminator
  Z Rate Transition : RateTransition  Deterministic=off  OutPortSampleTime=50E-3
  Out1 : Outport
  Out2 : Outport  Port=2
  Out3 : Outport  Port=3
  wires:
  Demux/7 -> Z Rate Transition/1
  In1/1 -> Demux/1
  Demux/1 -> Roll Rate Transition/1
  Demux/2 -> Terminator1/1
  Demux/3 -> Pitch Rate Transition/1
  Demux/4 -> Terminator3/1
  Demux/5 -> Terminator4/1
  Demux/6 -> Terminator5/1
  Demux/9 -> Terminator7/1
  Demux/10 -> Terminator8/1
  Demux/11 -> Terminator14/1
  Demux/12 -> Terminator12/1
  Demux/8 -> Terminator6/1
  Roll Rate Transition/1 -> Out1/1
  Pitch Rate Transition/1 -> Out2/1
  Z Rate Transition/1 -> Out3/1

== system systema2011a/CONTROL/RATE TRANSITION OUT ==
  In1 : Inport
  Rate Transition1 : RateTransition  Deterministic=off
  Out1 : Outport
  wires:
  In1/1 -> Rate Transition1/1
  Rate Transition1/1 -> Out1/1

== system systema2011a/CONTROL/Subsystem ==
  In1 : Inport
  Demux1 : Demux  Outputs=12
  Double click on this for demo.5 : Subsystem
      settings: OpenFcn=optsiminit
      mask Display: disp('optsiminit')
  Mux1 : Mux  Inputs=10
  Out2 : Outport
  Out3 : Outport  Port=2
  Out4 : Outport  Port=3
  wires:
  Demux1/1 -> Mux1/1
  Demux1/2 -> Mux1/2
  Demux1/3 -> Mux1/3
  Demux1/4 -> Mux1/4
  Demux1/5 -> Mux1/5
  Demux1/6 -> Mux1/6
  Demux1/7 -> Mux1/7
  Demux1/8 -> Mux1/8
  Demux1/10 -> Mux1/9
  Demux1/12 -> Mux1/10
  Mux1/1 -> Out2/1
  Demux1/9 -> Out3/1
  Demux1/11 -> Out4/1
  In1/1 -> Demux1/1

== system systema2011a/CONTROL/Subsystem1 ==
  In1 : Inport
  In2 : Inport  Port=2
  In3 : Inport  Port=3
  Demux1 : Demux  Outputs=10
  Mux1 : Mux  Inputs=12
  Out5 : Outport
  wires:
  In1/1 -> Demux1/1
  Demux1/1 -> Mux1/1
  Demux1/2 -> Mux1/2
  Demux1/3 -> Mux1/3
  Demux1/4 -> Mux1/4
  Demux1/5 -> Mux1/5
  Demux1/6 -> Mux1/6
  Demux1/7 -> Mux1/7
  Demux1/8 -> Mux1/8
  Demux1/10 -> Mux1/12
  Demux1/9 -> Mux1/10
  In2/1 -> Mux1/9
  In3/1 -> Mux1/11
  Mux1/1 -> Out5/1

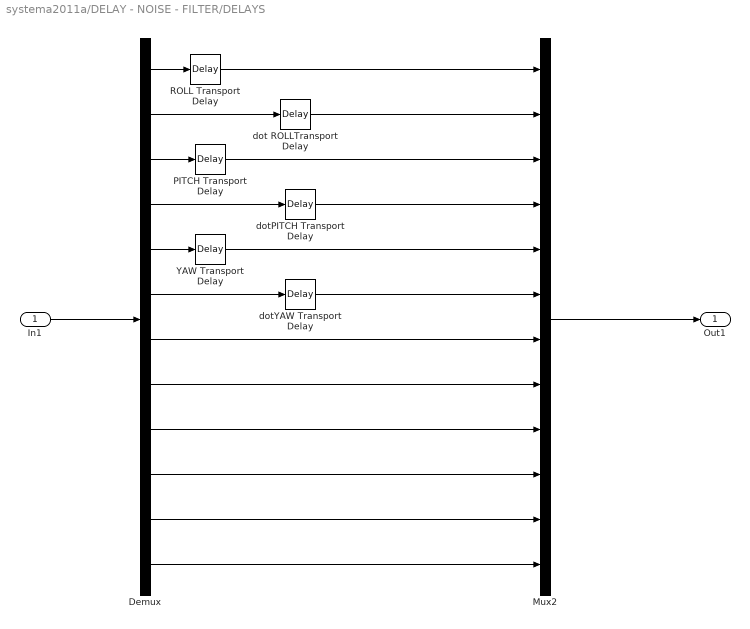
== system systema2011a/DELAY - NOISE - FILTER/DELAYS ==
  In1 : Inport
  Demux : Demux  Outputs=12
  Mux2 : Mux  Inputs=12
  PITCH Transport Delay : TransportDelay  DelayTime=8E-3
  ROLL Transport Delay : TransportDelay  DelayTime=8E-3
  YAW Transport Delay : TransportDelay  DelayTime=8E-3
  dot ROLLTransport Delay : TransportDelay  DelayTime=4.5E-3
  dotPITCH Transport Delay : TransportDelay  DelayTime=4.5E-3
  dotYAW Transport Delay : TransportDelay  DelayTime=4.5E-3
  Out1 : Outport
  wires:
  dot ROLLTransport Delay/1 -> Mux2/2
  Demux/12 -> Mux2/12
  Demux/11 -> Mux2/11
  Demux/10 -> Mux2/10
  Demux/9 -> Mux2/9
  Demux/8 -> Mux2/8
  Demux/7 -> Mux2/7
  dotYAW Transport Delay/1 -> Mux2/6
  Demux/6 -> dotYAW Transport Delay/1
  YAW Transport Delay/1 -> Mux2/5
  Demux/5 -> YAW Transport Delay/1
  dotPITCH Transport Delay/1 -> Mux2/4
  Demux/4 -> dotPITCH Transport Delay/1
  PITCH Transport Delay/1 -> Mux2/3
  Demux/3 -> PITCH Transport Delay/1
  Demux/2 -> dot ROLLTransport Delay/1
  ROLL Transport Delay/1 -> Mux2/1
  Demux/1 -> ROLL Transport Delay/1
  In1/1 -> Demux/1
  Mux2/1 -> Out1/1

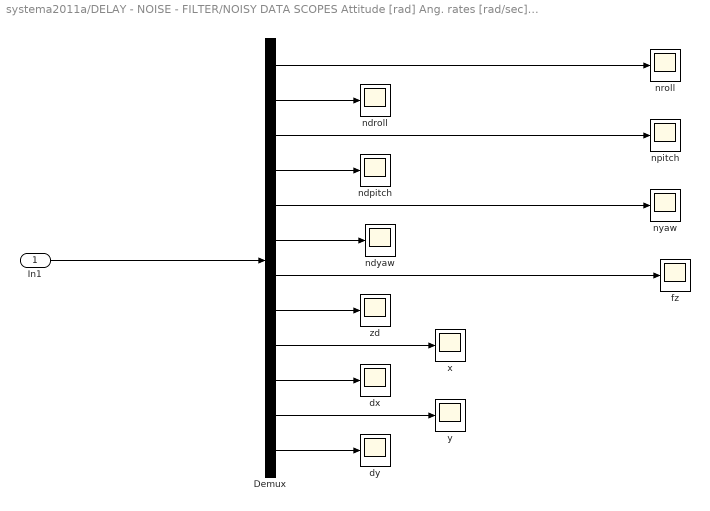
== system systema2011a/DELAY - NOISE - FILTER/NOISY DATA SCOPES Attitude [rad] Ang. rates [rad/sec] position [m] Pos. rates [m/s]1 ==
  In1 : Inport
  Demux : Demux  Outputs=12
  dx : Scope
      settings: TimeRange=5  MaxDataPoints=5000  SaveToWorkspace=off  SaveName=ScopeData5  YMin=0  YMax=0.009  SampleTime=-1
  dy : Scope
      settings: TimeRange=5  MaxDataPoints=5000  SaveToWorkspace=off  SaveName=ScopeData10  YMin=0  YMax=0.009  SampleTime=-1
  fz : Scope
      settings: TimeRange=5  MaxDataPoints=5000  SaveToWorkspace=off  SaveName=ScopeData17  YMin=0  YMax=0.009  SampleTime=-1
  ndpitch : Scope
      settings: TimeRange=auto  MaxDataPoints=5000  SaveToWorkspace=off  SaveName=ScopeData15  YMin=-2250  YMax=2250  SampleTime=-1
  ndroll : Scope
      settings: TimeRange=auto  MaxDataPoints=5000  SaveToWorkspace=off  SaveName=ScopeData14  YMin=-0.25  YMax=-0.05  SampleTime=-1
  ndyaw : Scope
      settings: TimeRange=18  MaxDataPoints=5000  SaveToWorkspace=off  SaveName=ScopeData16  YMin=-200  YMax=200  SampleTime=-1
  npitch : Scope
      settings: TimeRange=4  MaxDataPoints=5000  SaveToWorkspace=off  YMin=-1  YMax=1  SampleTime=-1
  nroll : Scope
      settings: TimeRange=0.25  MaxDataPoints=5000  SaveToWorkspace=off  SaveName=ScopeData  YMin=-1  YMax=1  SampleTime=-1
  nyaw : Scope
      settings: TimeRange=5  MaxDataPoints=5000  SaveToWorkspace=off  SaveName=ScopeData2  YMin=0  YMax=0.22  SampleTime=-1
  x : Scope
      settings: TimeRange=5  MaxDataPoints=5000  SaveToWorkspace=off  SaveName=ScopeData4  YMin=0  YMax=0.009  SampleTime=-1
  y : Scope
      settings: TimeRange=5  MaxDataPoints=5000  SaveToWorkspace=off  SaveName=ScopeData6  YMin=0  YMax=0.009  SampleTime=-1
  zd : Scope
      settings: TimeRange=10  MaxDataPoints=5000  SaveToWorkspace=off  SaveName=ScopeData18  YMin=-110.5  YMax=-107.25  SampleTime=-1
  wires:
  Demux/1 -> nroll/1
  Demux/4 -> ndpitch/1
  Demux/8 -> zd/1
  Demux/7 -> fz/1
  Demux/6 -> ndyaw/1
  Demux/2 -> ndroll/1
  Demux/5 -> nyaw/1
  Demux/3 -> npitch/1
  In1/1 -> Demux/1
  Demux/9 -> x/1
  Demux/10 -> dx/1
  Demux/11 -> y/1
  Demux/12 -> dy/1

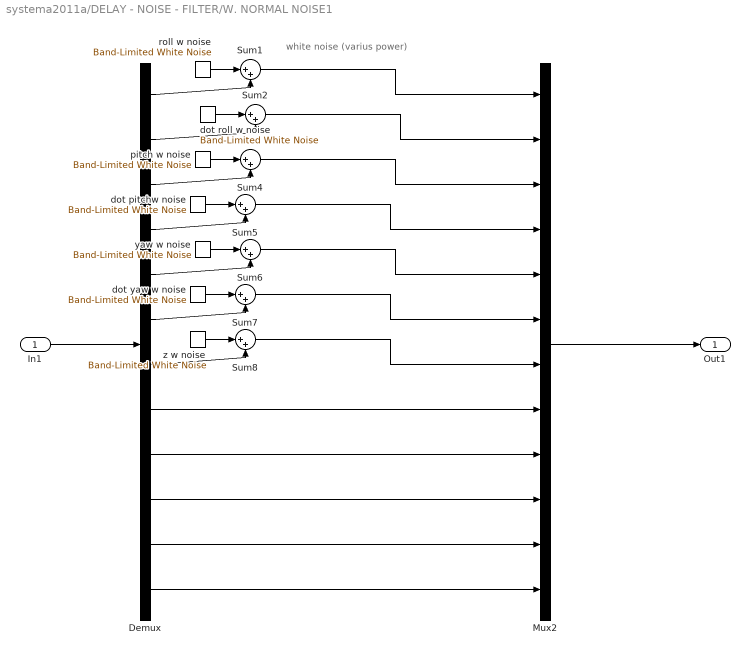
== system systema2011a/DELAY - NOISE - FILTER/W. NORMAL NOISE1 ==
  note: white noise (varius power)
  In1 : Inport
  Demux : Demux  Outputs=12
  Mux2 : Mux  Inputs=12
  Sum{1..2,4..8} (7 alike) : Sum  Inputs=|++  SaturateOnIntegerOverflow=on
  dot pitchw noise : simulink/Sources/Band-Limited White Noise  Cov=[0.0001]  Ts=0.01  seed=[23341]
  dot roll w noise : simulink/Sources/Band-Limited White Noise  Cov=[0.0001]  Ts=0.01  seed=[23341]
  dot yaw w noise : simulink/Sources/Band-Limited White Noise  Cov=[0.0001]  Ts=0.01  seed=[23341]
  pitch w noise : simulink/Sources/Band-Limited White Noise  Cov=[0.00001]  Ts=0.01  seed=[23341]
  roll w noise : simulink/Sources/Band-Limited White Noise  Cov=[0.00001]  Ts=0.01  seed=[24431]
  yaw w noise : simulink/Sources/Band-Limited White Noise  Cov=[0.00001]  Ts=0.01  seed=[23341]
  z w noise : simulink/Sources/Band-Limited White Noise  Cov=[0.00001]  Ts=0.01  seed=[23341]
  Out1 : Outport
  wires:
  Demux/8 -> Mux2/8
  Demux/12 -> Mux2/12
  Demux/11 -> Mux2/11
  Demux/10 -> Mux2/10
  Demux/9 -> Mux2/9
  Sum8/1 -> Mux2/7
  z w noise/1 -> Sum8/1
  Demux/7 -> Sum8/2
  Sum7/1 -> Mux2/6
  dot yaw w noise/1 -> Sum7/1
  Demux/6 -> Sum7/2
  Sum6/1 -> Mux2/5
  yaw w noise/1 -> Sum6/1
  Demux/5 -> Sum6/2
  Sum5/1 -> Mux2/4
  dot pitchw noise/1 -> Sum5/1
  Demux/4 -> Sum5/2
  Sum4/1 -> Mux2/3
  pitch w noise/1 -> Sum4/1
  Demux/3 -> Sum4/2
  Sum2/1 -> Mux2/2
  dot roll w noise/1 -> Sum2/1
  Demux/2 -> Sum2/2
  Sum1/1 -> Mux2/1
  roll w noise/1 -> Sum1/1
  Mux2/1 -> Out1/1
  In1/1 -> Demux/1
  Demux/1 -> Sum1/2

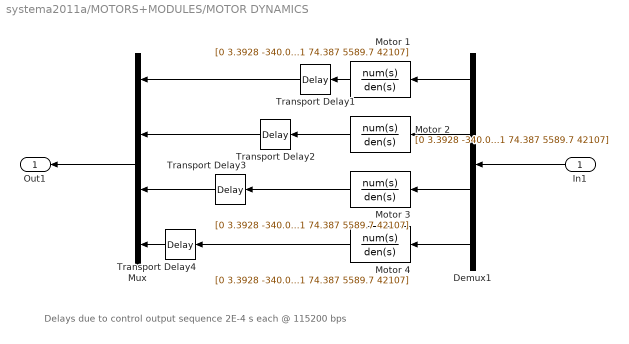
== system systema2011a/MOTORS+MODULES/MOTOR DYNAMICS ==
  note: Delays due to control output sequence
      | 2E-4 s each @ 115200 bps
  In1 : Inport
  Demux1 : Demux
  Motor {1..4} (4 alike) : TransferFcn  Numerator=[0 3.3928 -340.09 39451]  Denominator=[1 74.387 5589.7 42107]
  Mux : Mux
  Transport Delay1 : TransportDelay  DelayTime=2E-4
  Transport Delay2 : TransportDelay  DelayTime=4E-4
  Transport Delay3 : TransportDelay  DelayTime=6E-4
  Transport Delay4 : TransportDelay  DelayTime=8E-4
  Out1 : Outport
  wires:
  In1/1 -> Demux1/1
  Demux1/1 -> Motor 1/1
  Demux1/2 -> Motor 2/1
  Demux1/3 -> Motor 3/1
  Demux1/4 -> Motor 4/1
  Motor 1/1 -> Transport Delay1/1
  Motor 2/1 -> Transport Delay2/1
  Motor 3/1 -> Transport Delay3/1
  Motor 4/1 -> Transport Delay4/1
  Mux/1 -> Out1/1
  Transport Delay2/1 -> Mux/2
  Transport Delay3/1 -> Mux/3
  Transport Delay4/1 -> Mux/4
  Transport Delay1/1 -> Mux/1

== system systema2011a/Subsystem/Double click on this for demo.5 ==

== system systema2011a/CONTROL/Subsystem/Double click on this for demo.5 ==
